simulink model "Compare_Blockslx"  (R2023a)
settings: Solver=VariableStepAuto  StartTime=0.0  StopTime=10.0  RelTol=1e-3
libraries: simulink x4
settings Model: Creator=Aman  LastModifiedBy=Aman

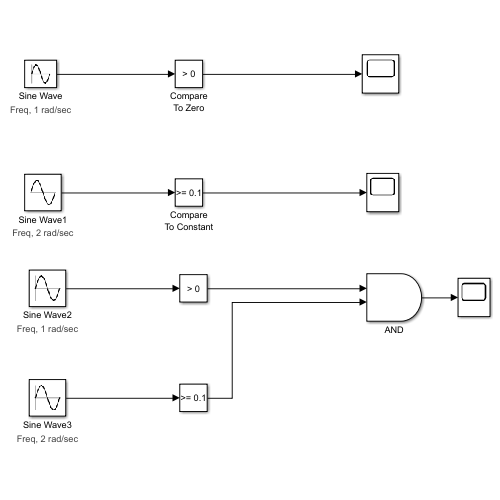
[thumbnail: Simulink's stored preview of the top-level diagram]
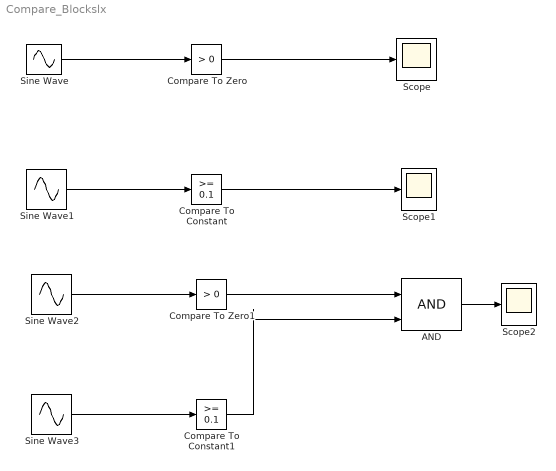
== system Compare_Blockslx ==
  AND : Logic  IconShape=distinctive  AllPortsSameDT=off  OutDataTypeStr=boolean
  Compare To Constant : simulink/Logic and Bit Operations/Compare To Constant  relop=>=  const=0.1  OutDataTypeStr=boolean
  Compare To Constant1 : simulink/Logic and Bit Operations/Compare To Constant  relop=>=  const=0.1  OutDataTypeStr=boolean
  Compare To Zero : simulink/Logic and Bit Operations/Compare To Zero  relop=>  OutDataTypeStr=boolean
  Compare To Zero1 : simulink/Logic and Bit Operations/Compare To Zero  relop=>  OutDataTypeStr=boolean
  Scope : Scope
  Scope1 : Scope
  Scope2 : Scope
  Sine Wave : Sin  SampleTime=0
      settings: AttributesFormatString=Freq, %<Frequency> rad/sec
  Sine Wave1 : Sin  Frequency=2  SampleTime=0
      settings: AttributesFormatString=Freq, %<Frequency> rad/sec
  Sine Wave2 : Sin  SampleTime=0
      settings: AttributesFormatString=Freq, %<Frequency> rad/sec
  Sine Wave3 : Sin  Frequency=2  SampleTime=0
      settings: AttributesFormatString=Freq, %<Frequency> rad/sec
  wires:
  Sine Wave/1 -> Compare To Zero/1
  Compare To Zero/1 -> Scope/1
  Sine Wave1/1 -> Compare To Constant/1
  Compare To Constant/1 -> Scope1/1
  Sine Wave3/1 -> Compare To Constant1/1
  Compare To Zero1/1 -> AND/1
  Compare To Constant1/1 -> AND/2
  AND/1 -> Scope2/1
  Sine Wave2/1 -> Compare To Zero1/1
